simulink model "io304"  (Simulink 6.0)
settings: Solver=ode5  StartTime=0.0  StopTime=10.0  RelTol=1e-3
libraries: xpclib x2
settings Model: Creator=ekbas  LastModifiedBy=ekbas  ExtModeArmWhenConnect=off
settings DataIOCC: SaveFormat=Structure  SignalLoggingName=sigsOut
settings DebuggingCC: CheckExecutionContextPreStartOutputMsg=on  CheckExecutionContextRuntimeOutputMsg=on  SolverPrmCheckMsg=none
settings RTWCC: SystemTargetFile=xpctarget.tlc  TemplateMakefile=xpc_default_tmf  Description=xPC Target  ProcessScript=xpctarget_make_rtw_hook
settings xpcTargetCC: TargetFcnLib=ansi_tfl_tmw.mat  GenFloatMathFcnCalls=ANSI_C  MatFileLogging=off
settings SFSimCC: SFSimApplyToAllLibs=on  SFSimBuildMode=Incremental

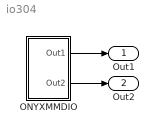
== system io304 ==
  ONYXMMDIO : Subsystem  PropExecContextAcrossSSBoundary=on
  Out1 : Outport
  Out2 : Outport  Port=2
  wires:
  ONYXMMDIO/1(Out1) -> Out1/1
  ONYXMMDIO/2(Out2) -> Out2/1

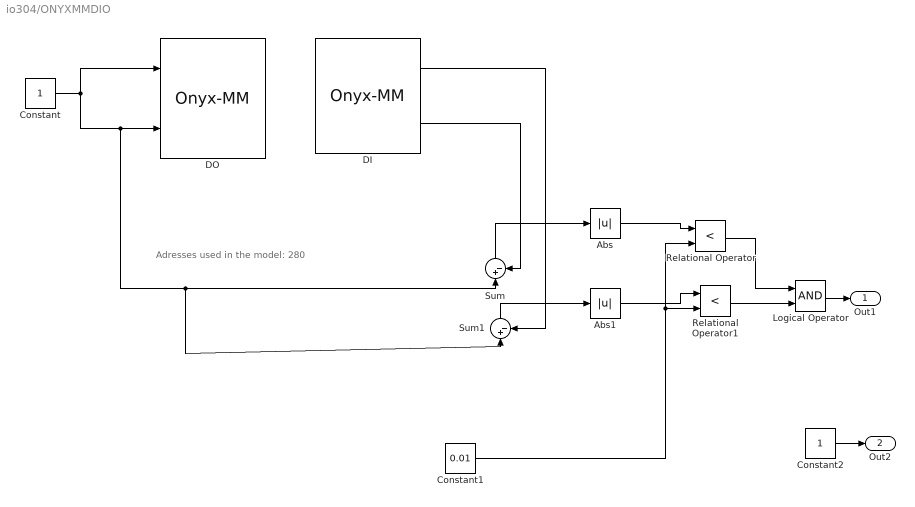
== system io304/ONYXMMDIO ==
  note: Adresses used in the model: 280
  Abs : Abs  SaturateOnIntegerOverflow=on
  Abs1 : Abs  SaturateOnIntegerOverflow=on
  Constant : Constant
  Constant1 : Constant  Value=0.01
  Constant2 : Constant
  DI : xpclib/Digital Input/Diamond/Onyx-MM   channel=[1 5]  port=B  chip=1  sampletime=.001  baseaddress=0x240
  DO : xpclib/Digital Output/Diamond/Onyx-MM   channel=[1 5]  port=C  reset=[1]  initValue=[0]  chip=1  sampletime=.001  baseaddress=0x240
  Logical Operator : Logic  AllPortsSameDT=off
  Relational Operator : RelationalOperator  Operator=<
  Relational Operator1 : RelationalOperator  Operator=<
  Sum : Sum  Orientation=up  Inputs=|+-  SaturateOnIntegerOverflow=on
  Sum1 : Sum  Orientation=up  Inputs=|+-  SaturateOnIntegerOverflow=on
  Out1 : Outport
  Out2 : Outport  Port=2
  wires:
  Abs1/1 -> Relational Operator1/1
  Constant1/1 -> Relational Operator/2, Relational Operator1/2
  DI/2 -> Sum/2
  DI/1 -> Sum1/2
  Relational Operator/1 -> Logical Operator/1
  Abs/1 -> Relational Operator/1
  Sum1/1 -> Abs1/1
  Sum/1 -> Abs/1
  Constant/1 -> Sum1/1, Sum/1, DO/2, DO/1
  Relational Operator1/1 -> Logical Operator/2
  Logical Operator/1 -> Out1/1
  Constant2/1 -> Out2/1
